simulink model "missileSystem"  (R2014a)
settings: Solver=ode45  StartTime=0.0  StopTime=10.0  RelTol=1e-3
undefined symbols (not defined in the file or in its folder): Arb, Brb, Crb, Drb, tau_act
settings Model: Creator=s220385  LastModifiedBy=s220385

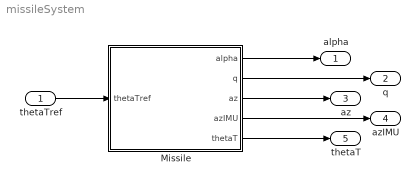
== system missileSystem ==
  thetaTref : Inport
  Missile : Subsystem  TreatAsAtomicUnit=on
      settings: MinAlgLoopOccurrences=on
      mask Display:
      | port_label('input', 1, '\theta_{Tref}','texmode','on')
      | 
      | port_label('output', 1, '\alpha','texmode','on')
      | port_label('output', 2, 'q','texmode','on')
      | port_label('output', 3, 'a_z','texmode','on')
      | port_label('output', 4, 'a_{zIMU}','texmode','on')
      | port_label('output', 5, '\theta_T','texmode','on')
  alpha : Outport
  q : Outport  Port=2
  az : Outport  Port=3
  azIMU : Outport  Port=4
  thetaT : Outport  Port=5
  wires:
  thetaTref/1 -> Missile/1(thetaTref)
  Missile/1(alpha) -> alpha/1
  Missile/3(az) -> az/1
  Missile/5("thetaT ") -> thetaT/1
  Missile/2(q) -> q/1
  Missile/4(azIMU) -> azIMU/1

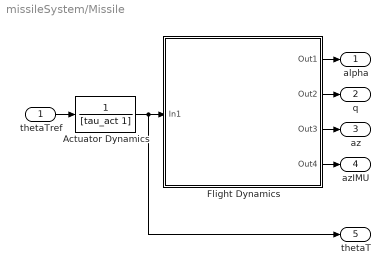
== system missileSystem/Missile ==
  thetaTref : Inport
  Actuator Dynamics : TransferFcn  Denominator=[tau_act 1]
  Flight Dynamics : Subsystem  TreatAsAtomicUnit=on
      settings: MinAlgLoopOccurrences=on
      mask Display:
      | port_label('input', 1, '\theta_T','texmode','on')
      | 
      | port_label('output', 1, '\alpha','texmode','on')
      | port_label('output', 2, 'q','texmode','on')
      | port_label('output', 3, 'a_z','texmode','on')
      | port_label('output', 4, 'a_{zIMU}','texmode','on')
  alpha : Outport
  q : Outport  Port=2
  az : Outport  Port=3
  azIMU : Outport  Port=4
  "thetaT " : Outport  Port=5
  wires:
  thetaTref/1 -> Actuator Dynamics/1
  Flight Dynamics/4(Out4) -> azIMU/1
  Flight Dynamics/2(Out2) -> q/1
  Flight Dynamics/1(Out1) -> alpha/1
  Actuator Dynamics/1 -> "thetaT "/1, Flight Dynamics/1(In1)
  Flight Dynamics/3(Out3) -> az/1

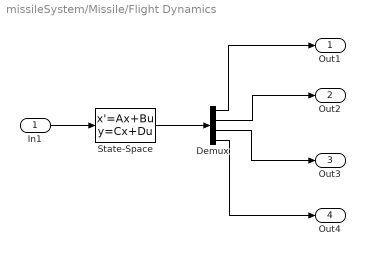
== system missileSystem/Missile/Flight Dynamics ==
  In1 : Inport
  Demux : Demux
  State-Space : StateSpace  A=Arb  B=Brb  C=Crb  D=Drb  X0=0
  Out1 : Outport
  Out2 : Outport  Port=2
  Out3 : Outport  Port=3
  Out4 : Outport  Port=4
  wires:
  In1/1 -> State-Space/1
  State-Space/1 -> Demux/1
  Demux/3 -> Out3/1
  Demux/2 -> Out2/1
  Demux/4 -> Out4/1
  Demux/1 -> Out1/1
